simulink model "GFM_L_Filter_cc"  (R2016a)
settings: Solver=ode23tb  SolverMode=SingleTasking  StartTime=0.0  StopTime=Simulation_Time  FixedStep=Time_Step2  MaxStep=1e-5  RelTol=1e-3
PreLoadFcn:
  | GFM_L_Filter_Init;
InitFcn:
  | GFM_L_Filter_Init;
undefined symbols (not defined in the file): Chosen_Strategy, dur1, dur2, egfault, fb, GRD00_Lg, GRD00_Rg, Ib2, kd, Ki_cc_cp, Ki_Inertia_Less, Kp_cc_cp, kp_GFo, Kp_Inertia_Less, R, Sb, Start, Theta_Vvsc0, Time_Step, Time_Step2, Ug, Va0, Vb0, Vb1, Vb2, Vc0, Vm0, Vvsc0, wb, Zb
libraries: powerlib x25, Control_Lib x14, simulink x5, Source_Lib x1
(part 1 of 2)
settings Model: Creator=Frederic_Colas  LastModifiedBy=Frederic_Colas
settings DebuggingCC: UnconnectedInputMsg=none  UnconnectedOutputMsg=none  UnconnectedLineMsg=none  SFUnexpectedBacktrackingDiag=error  SFNoUnconditionalDefaultTransitionDiag=error
settings HardwareCC: ProdWordSize=32  ProdHWDeviceType=Specified
settings GRTTargetCC: TargetLangStandard=C99 (ISO)
settings ConfigComp: CovMetricSettings=dwe  CovSaveCumulativeToWorkspaceVar=off  CovSaveSingleToWorkspaceVar=off  CovExternalEMLEnable=on
settings SimscapeCC: SimscapeNormalizeSystem=off

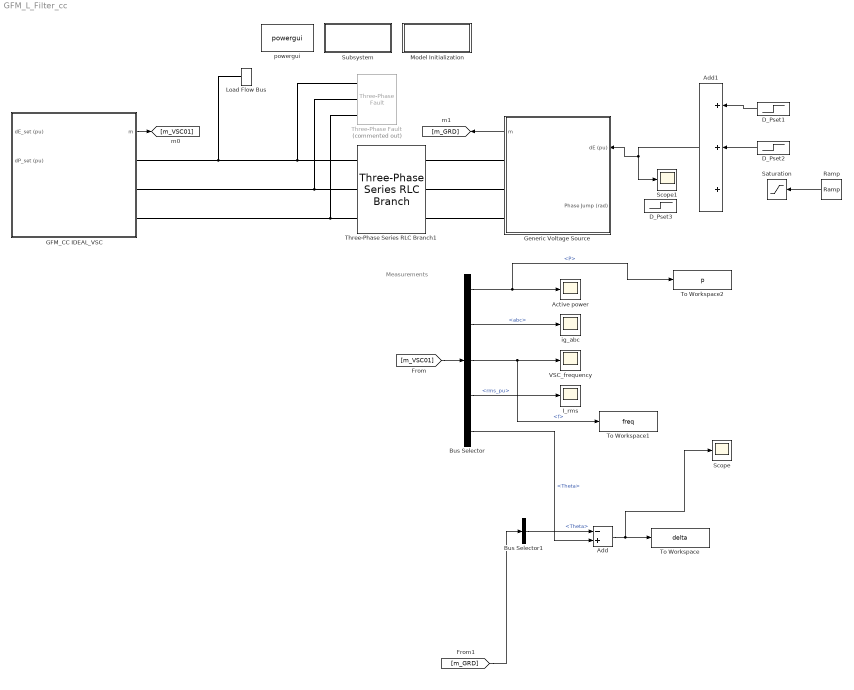
== system GFM_L_Filter_cc ==
  note: Measurements
  Active power : Scope
  Add : Sum  Inputs=-+
  Add1 : Sum  Inputs=+++
  Bus Selector : BusSelector  OutputSignals=P,Ig.abc,f,Ig.rms_pu,Theta
  Bus Selector1 : BusSelector  OutputSignals=Theta.Theta
  D_Pset1 : Step  Time=Start+0.1  After=-(1-egfault)  SampleTime=0
  D_Pset2 : Step  Time=Start+dur1+0.1  After=(1-egfault)  SampleTime=0
  D_Pset3 : Step  After=pi/6  SampleTime=0
  GFM_CC IDEAL_VSC : Subsystem  mask(VSC){fn=50, Sn=1000e6, Pn=1000e6, Udcn=640e3, Output_Delay=100e-6, Un1=320e3, Un2=400e3, Rt_pu=0.005, Lt_pu=0.15, Lm_pu=500, Rm_pu=500, DC_Link=Perfect DC Source, H_DC=inf, H_DC_sav=inf, wn_PLL=50, zeta_PLL=1, Val_Freq_Support=off, R_percent=4, dLc_pu=0.3, Rv=0.09, W_TVR=60, I_max_pu=1.2, Tr_I_max=10, Tau_fCC=0.01, wn_CC=1000, Kffi=on, Filtre_FF=off, w_ff=1000, Advanced=off, gainpopup=With Inertia, wn_Inertia_Less=5/(2*pi), Param_Inertia=PI, H_GFo=5, zeta_GFo=1, LFpopup=PV, P0=0.9, Q0=-0.069426, V0=1, Theta0=2.5991}
      mask prompts: fn "Nominal Frequency (Hz)"; Sn "Nominal Apparent Power (VA)"; Pn "Nominal Power (W)"; Udcn "Nominal DC Voltage (V)"; Output_Delay "Equivalent Output Delay (s)"; Un1 "VSC side Nominal Ph-Ph Voltage (V)"; Un2 "Grid side Nominal Ph-Ph Voltage (V)"; Rt_pu "R (pu)"; Lt_pu "L (pu)"; Lm_pu "Rm (pu)"; Rm_pu "Lm (pu)"; H_DC "DC inertia (ms)"; wn_PLL "Bandwidth (rad/s)"; zeta_PLL "Damping Ratio"; Val_Freq_Support "Frequency Support"; R_percent "Droop Gain (%)"; dLc_pu "Additional Virtual Impedance (pu)"; Rv "Damping Resistance (Rv)"; W_TVR "Dr filter"; I_max_pu "I max (pu)"; Tr_I_max "Current Loop time response (ms)"; Tau_fCC "Filter Time constant (s)"; wn_CC "Current Loop Bandwidth (rad/s))"; Kffi "Feedforward Enable"; Filtre_FF "Filter of ff enable"; w_ff "ff Filter Cutoff pulsation (rad/s)"; gainpopup "Strategy"; wn_Inertia_Less "Bandwidth (rad/s)"; H_GFo "Inertia H (s)"; zeta_GFo "Damping Ratio"; P0 "Initial Active Power (pu)"; Q0 "Initial Reactive Power (pu)"; V0 "Initial Voltage (pu)"; Theta0 "Initial Angle (°)"
      mask init:
      | Init_Base;
      | Init_VI;
      | Init_LF_L_modif;
      | Init_GFM_CC;
      settings: OpenFcn=|
      | NameStr = get_param(gcb,'Name');
      | open_system(gcbh, 'Mask');
      | 
      | h2AllOpenDlgs = DAStudio.ToolRoot.getOpenDialogs;
      | 
      | for i=1:length(h2AllOpenDlgs)
      |     try
      |          %disp(h2AllOpenDlgs(i).getSource.getBlock.Name);
      |         Dialog_block_name = h2AllOpenDlgs(i).getSource.getBlock.Name;
      |          %strcmp(Dialog_block_name, NameStr),
      |         if (strcmp(h2AllOpenDlgs(i).getSource.getBlock.Name, NameStr))
      |             iPos = h2AllOpenDlgs(i).position;
      |             h2AllOpenDlgs(i).position = [iPos(1)   iPos(2)   iPos(3)*1.4   iPos(4)];
      |         end
      |     end
      | end
      mask TypeOptions DC_Link: Perfect DC Source | No DC link capacitor | DC link capacitor
      mask Callback DC_Link:
      | % Get the mask parameter values. This is a cell
      | %   array of character vectors.
      | maskStr = get_param(gcb,'DC_Link');
      | p=Simulink.Mask.get(gcb);
      | 
      | % The pop-up menu is the first mask parameter.
      | %   Check the value selected in the pop-up
      | if strcmp(maskStr,'Perfect DC Source'),
      |     % Set the visibility of both parameters on when
      |     %   User-defined is selected in the pop-up.
      |     if strcmp(p.getParameter('H_DC').Visible,'on')
      |         p.getParameter('H_DC_sav').Value=p.getParameter('H_DC').Value;
      |     end
      |     p.getParameter('H_DC').Visible='off';
      |     p.getParameter('H_DC').Value='inf';
      | elseif strcmp(maskStr,'No DC link capacitor'),
      |     if strcmp(p.getParameter('H_DC').Visible,'on')
      |         p.getParameter('H_DC_sav').Value=p.getParameter('H_DC').Value;
      |     end
      |     p.getParameter('H_DC').Visible='off';
      |     p.getParameter('H_DC').Value='0';
      | else
      |     % Set the visibility of both parameters on when
      |     %   User-defined is selected in the pop-up.
      |     p.getParameter('H_DC').Visible='on';
      |     p.getParameter('H_DC').Value=p.getParameter('H_DC_sav').Value;
      | end
      mask Callback Advanced:
      | % Get the mask parameter values. This is a cell
      | %   array of character vectors.
      | maskStr = get_param(gcb,'Advanced');
      | p=Simulink.Mask.get(gcb);
      | 
      | % The pop-up menu is the first mask parameter.
      | %   Check the value selected in the pop-up
      | if strcmp(maskStr,'on'),
      | 
      |     % Set the visibility of both parameters on when
      |     %   User-defined is selected in the pop-up.
      |     %p.getDialogControl('TVR').Visible='on';
      |     %p.getDialogControl('TVI').Visible='on';
      |     %p.getDialogControl('LC_Filter').Visible='on';
      |     p.getDialogControl('Current_Sat').Visible='on';
      |     p.getDialogControl('CC').Visible='on';
      |     %p.getDialogControl('Param_Strat_3').Visible='off';
      | 
      | 
      | else
      | 
      |     % Set the visibility of both parameters on when
      |     %   User-defined is selected in the pop-up.
      |     %p.getDialogControl('TVR').Visible='off';
      |     %p.getDialogControl('TVI').Visible='off';
      |     %p.getDialogControl('LC_Filter').Visible='off';
      |     p.getDialogControl('Current_Sat').Visible='off';
      |     p.getDialogControl('CC').Visible='off';
      |     %p.getDialogControl('Param_Strat_3').Visible='off';
      | 
      | end
      mask TypeOptions gainpopup: Inertia Less | With Inertia
      mask Callback gainpopup:
      | % Get the mask parameter values. This is a cell
      | %   array of character vectors.
      | maskStr = get_param(gcb,'gainpopup');
      | p=Simulink.Mask.get(gcb);
      | 
      | % The pop-up menu is the first mask parameter.
      | %   Check the value selected in the pop-up
      | if strcmp(maskStr,'Inertia Less'),
      | 
      |     % Set the visibility of both parameters on when
      |     %   User-defined is selected in the pop-up.
      |     p.getDialogControl('No_Inertia').Visible='on';
      |     p.getDialogControl('Inertia').Visible='off';
      |     %p.getDialogControl('Param_Strat_3').Visible='off';
      | 
      | 
      | elseif strcmp(maskStr,'With Inertia'),
      | 
      |     % Set the visibility of both parameters on when
      |     %   User-defined is selected in the pop-up.
      |     p.getDialogControl('No_Inertia').Visible='off';
      |     p.getDialogControl('Inertia').Visible='on';
      |     %p.getDialogControl('Param_Strat_3').Visible='off';
      | 
      | 
      |     % Turn off the visibility of the Value field
      |     %   when User-defined is not selected.
      | 
      | else
      | 
      |     % Set the visibility of both parameters on when
      |     %   User-defined is selected in the pop-up.
      |     p.getDialogControl('No_Inertia').Visible='off';
      |     p.getDialogControl('Inertia').Visible='off';
      |     %p.getDialogControl('Param_Strat_3').Visible='off';
      | 
      | end
      mask TypeOptions Param_Inertia: VSM | PI
      mask TypeOptions LFpopup: Swing | PQ | PV
      mask Callback LFpopup:
      | % Get the mask parameter values. This is a cell
      | %   array of character vectors.
      | maskStr = get_param(gcb,'LFpopup');
      | p=Simulink.Mask.get(gcb);
      | 
      | % The pop-up menu is the first mask parameter.
      | %   Check the value selected in the pop-up
      | if strcmp(maskStr,'Swing'),
      | 
      |     % Set the visibility of both parameters on when
      |     %   User-defined is selected in the pop-up.
      |     p.getParameter('P0').Visible='off';
      |     p.getParameter('Q0').Visible='off';
      |     p.getParameter('V0').Visible='on';
      |     p.getParameter('Theta0').Visible='on';
      |     set_param([gcb '/Source_For_LF'],'BusType','swing');
      | 
      | elseif strcmp(maskStr,'PQ'),
      | 
      |     % Set the visibility of both parameters on when
      |     %   User-defined is selected in the pop-up.
      |     p.getParameter('P0').Visible='on';
      |     p.getParameter('Q0').Visible='on';
      |     p.getParameter('V0').Visible='off';
      |     p.getParameter('Theta0').Visible='off';
      |     set_param([gcb '/Source_For_LF'],'BusType','PQ');
      | 
      |     % Turn off the visibility of the Value field
      |     %   when User-defined is not selected.
      | else
      | 
      |     % Set the visibility of both parameters on when
      |     %   User-defined is selected in the pop-up.
      |     p.getParameter('P0').Visible='on';
      |     p.getParameter('Q0').Visible='off';
      |     p.getParameter('V0').Visible='on';
      |     p.getParameter('Theta0').Visible='off';
      |     set_param([gcb '/Source_For_LF'],'BusType','PV');
      | 
      | end
      mask DialogControl Container13 Prompt: PLL
      mask DialogControl Container14 Prompt: Frequency Support
      mask DialogControl VI Prompt: Virtual Impedance
      mask DialogControl TVR Prompt: Transient Virtual Resistor
      mask DialogControl Current_Sat Prompt: Current Limitation
      mask DialogControl CC Prompt: Current Loop
      mask DialogControl Control4 Prompt: Initial Operating Point
      mask DialogControl Container24 Prompt: VSC side
      mask DialogControl LF_vsc_str Prompt: V0 = 1.0552 pu, Angle = 25.2352°
      mask DialogControl Container25 Prompt: PCC
      mask DialogControl UpdateLoadflow Prompt: Update Loadflow
      mask DialogControl UpdateLoadflow Callback: LoadFlow_VSC
      mask Display:
      | x1=0.05;
      | y1=0.2;
      | %
      | plot([0.5 0.5]+x1,[0.97,0.8]-y1)
      | plot([0.5 0.32]+x1,[0.80 0.71]-y1)
      | plot([0.32 0.32]+x1,[0.80 0.52]-y1)
      | plot([0.32 0.5]+x1,[0.62 0.52]-y1)
      | plot([0.5 0.5]+x1,[0.52 0.35]-y1)
      | plot([0.45 0.5 0.43]+x1,[0.59 0.52 0.51]-y1)
      | %
      | plot([0.28 0.28]+x1,[0.74 0.58]-y1)
      | plot([0.28 0.20]+x1,[0.66 0.66]-y1)
      | %
      | plot([0.5 0.63]+x1,[0.84 0.84]-y1)
      | plot([0.63 0.63]+x1,[0.84 0.72]-y1)
      | plot([0.63 0.59]+x1,[0.72 0.65]-y1)
      | plot([0.63 0.67]+x1,[0.72 0.65]-y1)
      | plot([0.59 0.67]+x1,[0.65 0.65]-y1)
      | plot([0.63 0.63]+x1,[0.65 0.47]-y1)
      | plot([0.5 0.63]+x1,[0.47 0.47]-y1)
      | plot([0.58 0.67]+x1,[0.72 0.72]-y1)
      | %
      | color('blue')
      | text(0.3,0.10,'L-Filter GFM CC')
      | 
      | port_label('input',1,'\DeltaE (pu)','texmode','on');
      | port_label('input',2,'\DeltaP (pu)','texmode','on');
      | port_label('output',1,'m');
      | port_label('rconn',1,'A');
      | port_label('rconn',2,'B');
      | port_label('rconn',3,'C');
      | port_label('lconn',1,'+');
      | port_label('lconn',2,'-');
  Generic Voltage Source : Subsystem  AncestorBlock=Source_Lib/Generic Voltage Source  mask(GenericVoltageSource){SourceNature_str=INFINITE, fn=50, Sn=1e9, Un=Ug, H_s=5, DroopOnOff=on, R_percent=4, TN=1, TD=2, Time_Step=Time_Step, LFpopup=Swing, P0=-0.89593, Q0=0.11017, V0=1, Theta0=0}
      mask prompts: SourceNature_str "Nature of the voltage source"; fn "Nominal frequency fn [Hz]"; Sn "Nominal apparent power Sn [VA]"; Un "Nominal voltage Un [V RMS Ph2Ph]"; H_s "Inertia H [s]"; DroopOnOff "Frequency DROOP activation"; R_percent "Droop gain Kp [%]"; TN "Network time constant Lead [s]"; TD "Network time constant Lag [s]"; Time_Step "Output Delay (s)"; P0 "Active power P0 (pu)"; Q0 "Reactive power Q0 (pu)"; V0 "Initial Voltage (pu)"; Theta0 "Initial angle (°)"
      mask init:
      | % Update Name of LF bus for internal purpose
      | NameStr = [get_param(gcb,'Name')];% '_LF'];
      | set_param([gcb '/Load Flow Bus'],'ID',NameStr);  
      | 
      | % Base specification
      | fb = fn;                % [Hz] base frequency
      | Sb = Sn;                % [VA] base power
      | Ub = Un;                % [V] base ph2ph voltage
      | Vb = Un/sqrt(3);        % [V] base ph2N voltage
      | Ib = Sb/(3*Vb);         % [A] base current
      | Zb = Vb*Ib;             % [Ohm] base impedance
      | 
      | % Set the frequency droop gain
      | R = R_percent / 100;
      | 
      | %Initialize correctly the LoadFlow bus parameters connected to PCC
      |     VLF = V0;
      |     ThetaLF = Theta0;
      |     if (LFpopup == 'PQ')
      |         VLF = 1;
      |         ThetaLF = 0;
      |     elseif (LFpopup == 'PV')
      |         VLF = V0;
      |         ThetaLF = 0;        
      |     end
      |     set_param([gcb '/Load Flow Bus'],'Vref',num2str(VLF),'Vangle',num2str(ThetaLF));
      | 
      | 
      | % Update mask display:
      | % mo = get_param(gcb,'MaskObject');
      | % Generate string to display LF results on Mask
      |     mo = get_param(gcb,'MaskObject');
      |     mo.getDialogControl('LF_pcc_str').Prompt = ['V0 = ', num2str(V0),' pu, Angle = ', num2str(Theta0),'°'];
      |     mo.getDialogControl('LF_pcc_Power_str').Prompt = ['P0 = ', num2str(P0),' pu, Q0 = ', num2str(Q0),' pu'];
      mask TypeOptions SourceNature_str: INFINITE | INERTIAL
      mask Callback SourceNature_str:
      | % Get the mask parameter values. This is a cell
      | %   array of character vectors.
      | maskStr = get_param(gcb,'SourceNature_str');
      | p=Simulink.Mask.get(gcb);
      | 
      | % The pop-up menu is the first mask parameter.
      | %   Check the value selected in the pop-up
      | if strcmp(maskStr,'INFINITE')
      |     p.getDialogControl('Inertial').Visible='off';
      |    %p.getParameter('H_s').Visible='off';
      |    %p.getParameter('DroopOnOff').Visible='off';
      |    %DroopOnOff = 'off';
      |    %p.getParameter('R_percent').Visible='off';
      |    %p.getParameter('TN').Visible='off';
      |    %p.getParameter('TD').Visible='off';
      |    set_param([gcb '/SourceNature'],'Value','1')
      | else
      |    %p.getParameter('H_s').Visible='on';
      |    %p.getParameter('DroopOnOff').Visible='on';
      |    %DroopOnOff = 'on';
      |    %p.getParameter('R_percent').Visible='on';
      |    %p.getParameter('TN').Visible='on';
      |    %p.getParameter('TD').Visible='on';
      |    p.getDialogControl('Inertial').Visible='on';
      |    set_param([gcb '/SourceNature'],'Value','2')
      | end
      mask Callback DroopOnOff:
      | % Get the mask parameter values. This is a cell
      | %   array of character vectors.
      | maskStr = get_param(gcb,'DroopOnOff');
      | p=Simulink.Mask.get(gcb);
      | 
      | if strcmp(maskStr,'on'),
      |     p.getParameter('R_percent').Enabled='on';
      | else
      |     p.getParameter('R_percent').Enabled='off';
      | end
      mask TypeOptions LFpopup: Swing | PQ | PV
      mask Callback LFpopup:
      | % Get the mask parameter values. This is a cell
      | %   array of character vectors.
      | maskStr = get_param(gcb,'LFpopup');
      | p=Simulink.Mask.get(gcb);
      | 
      | % The pop-up menu is the first mask parameter.
      | %   Check the value selected in the pop-up
      | if strcmp(maskStr,'Swing'),
      | 
      |     % Set the visibility of both parameters on when
      |     %   User-defined is selected in the pop-up.
      |     p.getParameter('P0').Visible='off';
      |     p.getParameter('Q0').Visible='off';
      |     p.getParameter('V0').Visible='on';
      |     p.getParameter('Theta0').Visible='on';
      |     set_param([gcb '/Source_For_LF'],'BusType','swing');
      | 
      | elseif strcmp(maskStr,'PQ'),
      | 
      |     % Set the visibility of both parameters on when
      |     %   User-defined is selected in the pop-up.
      |     p.getParameter('P0').Visible='on';
      |     p.getParameter('Q0').Visible='on';
      |     p.getParameter('V0').Visible='off';
      |     p.getParameter('Theta0').Visible='off';
      |     set_param([gcb '/Source_For_LF'],'BusType','PQ');
      | 
      |     % Turn off the visibility of the Value field
      |     %   when User-defined is not selected.
      | else
      | 
      |     % Set the visibility of both parameters on when
      |     %   User-defined is selected in the pop-up.
      |     p.getParameter('P0').Visible='on';
      |     p.getParameter('Q0').Visible='off';
      |     p.getParameter('V0').Visible='on';
      |     p.getParameter('Theta0').Visible='off';
      |     set_param([gcb '/Source_For_LF'],'BusType','PV');
      | 
      | end
      mask DialogControl Control1 Prompt: Initial Operating Point
      mask DialogControl Container6 Prompt: PCC
      mask DialogControl Control4 Prompt: Update Loadflow
      mask DialogControl Control4 Callback: LoadFlow_VSC
      mask Display:
      | if (SourceNature_str == 1)
      |     image(imread('infinite.png'));
      |     color('blue')
      |     text(0.3,0.10,'Infinite bus')
      | else
      |     image(imread('inertia.png'));
      |     color('blue')
      |     text(0.3,0.10,'Inertia Emulation')
      | end
      | 
      | port_label('input',1,'\DeltaE (pu)','texmode','on');
      | port_label('input',2,'\Delta\theta (rad)','texmode','on');
      | port_label('output',1,'m');
      | port_label('rconn',1,'A');
      | port_label('rconn',2,'B');
      | port_label('rconn',3,'C');
  I_rms : Scope
  Load Flow Bus : powerlib/Measurements/Load Flow Bus  LConnTagsString=a  Phases=single  Connectors=on one side  ID=BUS_1  Vbase=Ug  Vref=1  Vangle=0  VLF=1  VLFb=1  VLFc=1  angleLF=2.599  angleLFb=0  angleLFc=0
  Model Initialization : Subsystem  mask(Model Functions){InitFcnX=GFM_L_Filter_Init;, prel=on, posl=off, inif=on, strf=off}
      mask prompts: InitFcnX "Initialisation"; prel "Preload Function"; posl "PostLoad Function"; inif "InitFcn"; strf "StartFcn"
      mask init:
      | currentBlock = gcb;
      | root = bdroot(currentBlock);
      | 
      | if ~strcmp(get_param(root,'BlockDiagramType'),'library')
      |     if prel==1
      |         set_param(root, 'PreLoadFcn', InitFcnX);
      |     else
      |         set_param(root, 'PreLoadFcn', '');
      |     end
      |     if inif==1
      |         set_param(root, 'InitFcn', InitFcnX);
      |     else
      |         set_param(root, 'InitFcn', '');
      |     end
      |     if strf==1
      |         set_param(root, 'StartFcn', InitFcnX);
      |     else
      |         set_param(root, 'StartFcn', '');
      |     end
      |     if posl==1
      |         set_param(root, 'PostLoadFcn', InitFcnX);
      |     else
      |         set_param(root, 'PostLoadFcn', '');
      |     end
      | end
      | 
      | pos = get_param(currentBlock, 'Position');
      | width = pos(3) - pos(1); height = pos(4) - pos(2);
      | txt = [ upper(root) '\n' '- InitFcn. . . . . '  get_param(root, 'InitFcn') ];
      settings: CopyFcn=set_param(gcb,'LinkStatus','none')
      mask Display:
      | %text(5, height*0.5, txt, 'horizontalAlignment', 'left', 'verticalAlignment', 'middle') ;
      | color('blue'),disp('Initialization Function\nParameters')
  Ramp : simulink/Sources/Ramp  slope=(1-egfault)/(dur2)  start=Start+dur1+0.1  X0=0
  Saturation : Saturate  UpperLimit=1-egfault  LowerLimit=0
  Scope : Scope
  Scope1 : Scope
  Subsystem : Subsystem
      settings: OpenFcn=LoadFlow_VSC
      mask Display: color('blue'),disp('Update Loadflow')
  Three-Phase Series RLC Branch1 : powerlib/Elements/Three-Phase Series RLC Branch  LConnTagsString=A|B|C  RConnTagsString=A|B|C  BranchType=RL  Resistance=GRD00_Rg  Inductance=GRD00_Lg  Capacitance=1e-6  Measurements=None
  Three-Phase Fault : powerlib/Elements/Three-Phase Fault  Commented=on  InitialStates=0  FaultA=on  FaultB=on  FaultC=on  GroundFault=on  SwitchTimes=[0.2 0.4]  External=off  SwitchStatus=NaN  FaultResistance=0.001  GroundResistance=0.01  SnubberResistance=1e6  SnubberCapacitance=inf  Measurements=None
  To Workspace : ToWorkspace  VariableName=delta  SaveFormat=Timeseries  SampleTime=Time_Step
  To Workspace1 : ToWorkspace  VariableName=freq  SaveFormat=Timeseries  SampleTime=Time_Step
  To Workspace2 : ToWorkspace  VariableName=p  SaveFormat=Timeseries  SampleTime=Time_Step
  VSC_frequency : Scope
  ig_abc : Scope
  powergui : powerlib/powergui  Priority=1  SimulationMode=Discrete  SampleTime=Time_Step2  frequency=60  Iterations=50  frequencyindice=50  Pbase=1000000000  ErrMax=1e-6  UnitsV=kV  UnitsW=MW  buscounter=0  FunctionMessages=off  echomessages=off  EnableUseOfTLC=off  CurrentSourceSwitches=off  DisableSnubberDevices=off  DisableRonSwitches=off  DisableVfSwitches=off  DisplayEquations=off  AutomaticDiscreteSolvers=off  SolverType=Tustin/Backward Euler (TBE)  Interpol=off  ExternalGateDelay=off  methode=off  Ts=100  x0status=blocks  SPID=on  SwTol=0  HookPort=off  NonlinearTolerance=1e-4  nMaxIteration=100  ContinueOnMaxIteration=off  RestoreLinks=warning  ResistiveCurrentMeasurement=off  Frange=[0:2:500]  Ylog=off  Xlog=on  ShowGrid=off  save=off  variable=ZData  structure=0  ZoomFFT=off  StartTime=0.0  cycles=1  DisplayStyle=1  fundamental=60  FreqAxis=off  MaxFrequency=1000  frequencyindicesteady=1  RmsSteady=1  display=off
  wires:
  [m_VSC01] -> Bus Selector/1
  Bus Selector/1 -> To Workspace2/1, Active power/1  "<P>"
  Bus Selector/4 -> I_rms/1  "<rms_pu>"
  Bus Selector/2 -> ig_abc/1  "<abc>"
  Bus Selector/3 -> VSC_frequency/1, To Workspace1/1  "<f>"
  GFM_CC IDEAL_VSC/1(m) -> [m_VSC01]
  Generic Voltage Source/1(m) -> [m_GRD]
  [m_GRD] -> Bus Selector1/1
  Bus Selector1/1 -> Add/1  "<Theta>"
  Bus Selector/5 -> Add/2  "<Theta>"
  Add/1 -> Scope/1, To Workspace/1
  D_Pset1/1 -> Add1/1
  Ramp/1 -> Saturation/1
  D_Pset2/1 -> Add1/2
  Add1/1 -> Generic Voltage Source/1(dE (pu)), Scope1/1
  connections:
  Load Flow Bus/LConn1 -- Three-Phase Fault/LConn1 -- Three-Phase Series RLC Branch1/LConn1 -- GFM_CC IDEAL_VSC/RConn1
  GFM_CC IDEAL_VSC/RConn3 -- Three-Phase Fault/LConn3 -- Three-Phase Series RLC Branch1/LConn3
  GFM_CC IDEAL_VSC/RConn2 -- Three-Phase Fault/LConn2 -- Three-Phase Series RLC Branch1/LConn2
  Generic Voltage Source/RConn1 -- Three-Phase Series RLC Branch1/RConn1
  Generic Voltage Source/RConn2 -- Three-Phase Series RLC Branch1/RConn2
  Generic Voltage Source/RConn3 -- Three-Phase Series RLC Branch1/RConn3

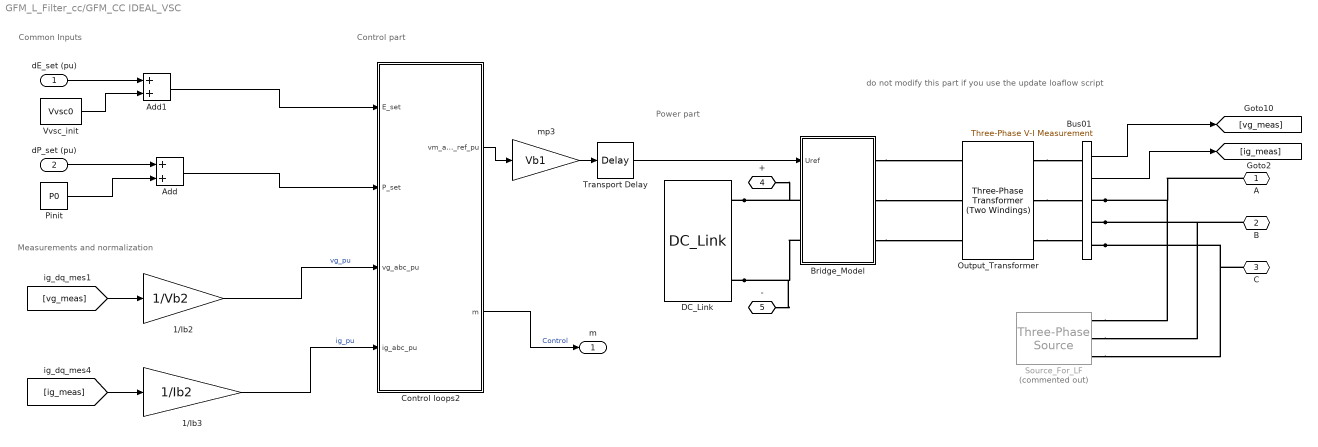
== system GFM_L_Filter_cc/GFM_CC IDEAL_VSC ==
  note: Control part
  note: Measurements and normalization
  note: Power part
  note: Common Inputs
  note: do not modify this part if you use the update loaflow script
  dE_set (pu) : Inport
  dP_set (pu) : Inport  Port=2
  1/Ib2 : Gain  Gain=1/Vb2
  1/Ib3 : Gain  Gain=1/Ib2
  Add : Sum
  Add1 : Sum
  Bridge_Model : Subsystem
  Bus01 : powerlib/Measurements/Three-Phase V-I Measurement  VoltageMeasurement=phase-to-ground  SetLabelV=off  LabelV=Vabc  Vpu=off  VpuLL=off  CurrentMeasurement=yes  SetLabelI=off  LabelI=Iabc  Ipu=off  Pbase=100e6  Vbase=500e3  OutputType=Complex  PhasorSimulation=off  PSBequivalent=0
  Control loops2 : Subsystem
  DC_Link : Source_Lib/DC_Link  Udc=Udcn  Pb=Pn  H_DC=H_DC
  Output_Transformer : powerlib/Elements/Three-Phase Transformer (Two Windings)  Winding1Connection=Yg  Winding2Connection=Yg  CoreType=Three single-phase transformers  SetSaturation=off  Hysteresis=off  DataFile='hysteresis'  SetInitialFlux=off  Measurements=None  UNITS=pu  NominalPower=[Sn , fb]  Winding1=[Un1 , Rt_pu/2 , Lt_pu/2]  Winding2=[Un2 , Rt_pu/2 , Lt_pu/2]  Rm=Rm_pu  Lm=Lm_pu  L0=0.5  Saturation=[ 0,0 ; 0.0024,1.2 ; 1.0,1.52 ]  InitialFluxes=[ 0.8 , -0.8 , 0.7 ]  BreakLoop=off  DiscreteSolver=Trapezoidal iterative  DataType=off  TransfoNumber=1
  Pinit : Constant  Value=P0
  Source_For_LF : powerlib/Electrical Sources/Three-Phase Source  Commented=on  InternalConnection=Yg  VoltagePhases=off  Voltage=(400000)*1  PhaseAngle=2.5991  Voltage_phases=[25e3 25e3 25e3]/sqrt(3)  PhaseAngles_phases=[0 -120 +120]  Frequency=fb  NonIdealSource=off  SpecifyImpedance=off  Resistance=0  Inductance=0  ShortCircuitLevel=100e6  BaseVoltage=Un  XRratio=7  BusType=PV  Pref=P0*Sb  Qref=Q0*Sb  Prefabc=[10e3, 10e3, 10e3]  Qrefabc=[0, 0, 0]  Qmin=-inf  Qmax=inf
  Transport Delay : TransportDelay  DelayTime=Output_Delay  InitialOutput=[Va0 Vb0 Vc0]
  Vvsc_init : Constant  Value=Vvsc0
  mp3 : Gain  Gain=Vb1
  A : PMIOPort  Side=Right
  B : PMIOPort  Port=2  Side=Right
  C : PMIOPort  Port=3  Side=Right
  + : PMIOPort  Port=4  Side=Left
  - : PMIOPort  Port=5  Side=Left
  m : Outport
  wires:
  [ig_meas] -> 1/Ib3/1
  Bus01/2 -> [ig_meas]
  dE_set (pu)/1 -> Add1/1
  Bus01/1 -> [vg_meas]
  Vvsc_init/1 -> Add1/2
  Pinit/1 -> Add/2
  dP_set (pu)/1 -> Add/1
  Transport Delay/1 -> Bridge_Model/1(Uref)
  Add1/1 -> Control loops2/1(E_set)
  Control loops2/1(vm_abc_ref_pu) -> mp3/1
  [vg_meas] -> 1/Ib2/1
  1/Ib2/1 -> Control loops2/3(vg_abc_pu)  "vg_pu"
  1/Ib3/1 -> Control loops2/4(ig_abc_pu)  "ig_pu"
  mp3/1 -> Transport Delay/1
  Control loops2/2(m) -> m/1  "Control"
  Add/1 -> Control loops2/2(P_set)
  connections:
  DC_Link/RConn3 -- -/RConn1 -- Bridge_Model/LConn2
  DC_Link/RConn1 -- +/RConn1 -- Bridge_Model/LConn1
  Bus01/RConn3 -- C/RConn1 -- Source_For_LF/RConn3
  Bus01/RConn1 -- A/RConn1 -- Source_For_LF/RConn1
  Bridge_Model/RConn3 -- Output_Transformer/LConn3
  Bridge_Model/RConn2 -- Output_Transformer/LConn2
  Bridge_Model/RConn1 -- Output_Transformer/LConn1
  Bus01/RConn2 -- B/RConn1 -- Source_For_LF/RConn2
  Output_Transformer/RConn3 -- Bus01/LConn3
  Output_Transformer/RConn2 -- Bus01/LConn2
  Output_Transformer/RConn1 -- Bus01/LConn1

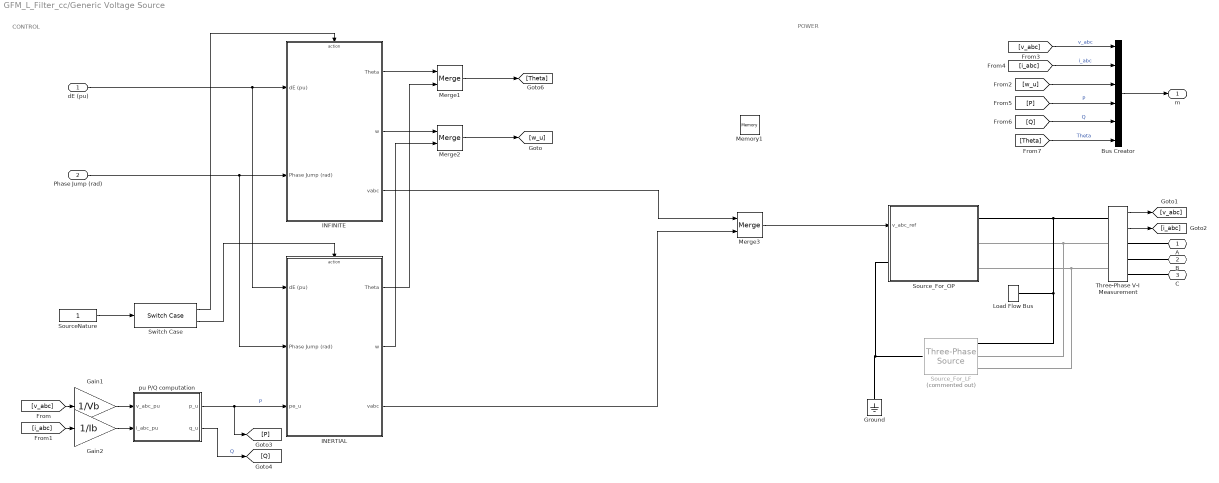
== system GFM_L_Filter_cc/Generic Voltage Source ==
  note: CONTROL
  note: POWER
  dE (pu) : Inport
  Phase Jump (rad) : Inport  Port=2
  " pu P/Q computation" : Subsystem  DialogController=POWERSYS.PowerSysDialog
  Bus Creator : BusCreator  Inputs=6
  Gain1 : Gain  Gain=1/Vb
  Gain2 : Gain  Gain=1/Ib
  Ground : powerlib/Elements/Ground  LConnTagsString=a
  INERTIAL : Subsystem
  INFINITE : Subsystem
  Load Flow Bus : powerlib/Measurements/Load Flow Bus  LConnTagsString=a  Phases=single  Connectors=on one side  ID=Generic Voltage Source  Vbase=Un  Vref=1  Vangle=0  VLF=1  VLFb=1  VLFc=1  angleLF=0  angleLFb=0  angleLFc=0
  Memory1 : Memory
  Merge1 : Merge
  Merge2 : Merge
  Merge3 : Merge
  SourceNature : Constant
  Source_For_LF : powerlib/Electrical Sources/Three-Phase Source  Commented=on  InternalConnection=Yn  VoltagePhases=off  Voltage=(400000)*1  PhaseAngle=0  Voltage_phases=[25e3 25e3 25e3]/sqrt(3)  PhaseAngles_phases=[0 -120 +120]  Frequency=fb  NonIdealSource=off  SpecifyImpedance=off  Resistance=0  Inductance=0  ShortCircuitLevel=100e6  BaseVoltage=Un  XRratio=7  BusType=swing  Pref=P0*Sb  Qref=Q0*Sb  Prefabc=[10e3, 10e3, 10e3]  Qrefabc=[0, 0, 0]  Qmin=-inf  Qmax=inf
  Source_For_OP : Subsystem
  Switch Case : SwitchCase  CaseConditions={1, 2}  ShowDefaultCase=off
  Three-Phase V-I Measurement : powerlib/Measurements/Three-Phase V-I Measurement  VoltageMeasurement=phase-to-ground  SetLabelV=off  LabelV=v_abc  Vpu=off  VpuLL=off  CurrentMeasurement=yes  SetLabelI=off  LabelI=i_abc  Ipu=off  Pbase=100e6  Vbase=500e3  OutputType=Complex  PhasorSimulation=off  PSBequivalent=0
  A : PMIOPort  Side=Right
  B : PMIOPort  Port=2  Side=Right
  C : PMIOPort  Port=3  Side=Right
  m : Outport
  wires:
  INERTIAL/3(vabc) -> Merge3/2
  INFINITE/3(vabc) -> Merge3/1
  Merge3/1 -> Source_For_OP/1(v_abc_ref)
  Merge2/1 -> [w_u]
  INERTIAL/2(w) -> Merge2/2
  INFINITE/2(w) -> Merge2/1
  INERTIAL/1(Theta) -> Merge1/2
  Phase Jump (rad)/1 -> INFINITE/2(Phase Jump (rad)), INERTIAL/2(Phase Jump (rad))
  dE (pu)/1 -> INFINITE/1(dE (pu)), INERTIAL/1(dE (pu))
  Merge1/1 -> [Theta]
  INFINITE/1(Theta) -> Merge1/1
  [Theta] -> Bus Creator/6  "Theta"
  SourceNature/1 -> Switch Case/1
  Switch Case/1 -> INFINITE/Action
  Switch Case/2 -> INERTIAL/Action
  [v_abc] -> Gain1/1
  [i_abc] -> Gain2/1
  Gain1/1 -> " pu P/Q computation"/1(v_abc_pu)
  Gain2/1 -> " pu P/Q computation"/2(i_abc_pu)
  " pu P/Q computation"/2(q_u) -> [Q]  "Q"
  " pu P/Q computation"/1(p_u) -> [P], INERTIAL/3(pe_u)  "P"
  [v_abc] -> Bus Creator/1  "v_abc"
  [i_abc] -> Bus Creator/2  "i_abc"
  [w_u] -> Bus Creator/3
  Bus Creator/1 -> m/1
  Three-Phase V-I Measurement/1 -> [v_abc]
  Three-Phase V-I Measurement/2 -> [i_abc]
  [P] -> Bus Creator/4  "P"
  [Q] -> Bus Creator/5  "Q"
  connections:
  Source_For_LF/RConn2 -- Three-Phase V-I Measurement/LConn2 -- Source_For_OP/RConn2
  Source_For_OP/LConn1 -- Ground/LConn1
  Source_For_LF/RConn3 -- Three-Phase V-I Measurement/LConn3 -- Source_For_OP/RConn3
  Source_For_OP/RConn1 -- Source_For_LF/RConn1 -- Load Flow Bus/LConn1 -- Three-Phase V-I Measurement/LConn1
  Three-Phase V-I Measurement/RConn1 -- A/RConn1
  Three-Phase V-I Measurement/RConn2 -- B/RConn1
  Three-Phase V-I Measurement/RConn3 -- C/RConn1

== system GFM_L_Filter_cc/Model Initialization ==

== system GFM_L_Filter_cc/Subsystem ==

== system GFM_L_Filter_cc/GFM_CC IDEAL_VSC/Bridge_Model ==
  Uref : Inport
  NOT1 : Logic  Operator=NOT  IconShape=distinctive  AllPortsSameDT=off  OutDataTypeStr=boolean
  Saturation : Saturate  UpperLimit=1  LowerLimit=-1
  Step : Step  Time=Output_Delay  SampleTime=0
  Three-Phase Breaker1 : powerlib/Elements/Three-Phase Breaker  InitialState=closed  SwitchA=on  SwitchB=on  SwitchC=on  SwitchTimes="[4/60  10/60]"  External=on  BreakerResistance=1e-5*Zb  SnubberResistance=1e6  SnubberCapacitance=inf  Measurements=None
  Three-Phase Breaker2 : powerlib/Elements/Three-Phase Breaker  InitialState=open  SwitchA=on  SwitchB=on  SwitchC=on  SwitchTimes="[4/60  10/60]"  External=on  BreakerResistance=1e-5*Zb  SnubberResistance=1e6  SnubberCapacitance=inf  Measurements=None
  Three-Phase Source : powerlib/Electrical Sources/Three-Phase Source  InternalConnection=Yg  VoltagePhases=off  Voltage=Vm0*Un1  PhaseAngle=Theta_Vm0  Voltage_phases=[25e3 25e3 25e3]/sqrt(3)  PhaseAngles_phases=[0 -120 +120]  Frequency=fb  NonIdealSource=off  SpecifyImpedance=off  Resistance=0  Inductance=0  ShortCircuitLevel=100e6  BaseVoltage=VSC01_Un1  XRratio=7  BusType=swing  Pref=0.3  Qref=0  Prefabc=[10e3, 10e3, 10e3]  Qrefabc=[0, 0, 0]  Qmin=-Inf  Qmax=Inf
  Universal Bridge : powerlib/Power Electronics/Universal Bridge  Arms=3  SnubberResistance=1e5  SnubberCapacitance=inf  Device=Average-model based VSC  Ron=1e-3  Lon=0  ForwardVoltages="[  0  0  ]"  ForwardVoltage=0  GTOparameters=[ 10e-6 , 20e-6 ]  IGBTparameters=[ 1e-6 , 2e-6 ]  Measurements=None  Measurements_2=None  converterType=Rectifier
  mp3 : Gain  Gain=2/Udcn
  PhA : PMIOPort  Side=Right
  PhB : PMIOPort  Port=2  Side=Right
  PhC : PMIOPort  Port=3  Side=Right
  Vdc+ : PMIOPort  Port=4  Side=Left
  Vdc- : PMIOPort  Port=5  Side=Left
  wires:
  Uref/1 -> mp3/1
  mp3/1 -> Saturation/1
  Step/1 -> NOT1/1, Three-Phase Breaker2/1
  NOT1/1 -> Three-Phase Breaker1/1
  Saturation/1 -> Universal Bridge/1
  connections:
  Universal Bridge/RConn2 -- Vdc-/RConn1
  Universal Bridge/RConn1 -- Vdc+/RConn1
  Three-Phase Source/RConn3 -- Three-Phase Breaker1/RConn3
  Three-Phase Source/RConn2 -- Three-Phase Breaker1/RConn2
  Three-Phase Source/RConn1 -- Three-Phase Breaker1/RConn1
  Three-Phase Breaker2/RConn3 -- Universal Bridge/LConn3
  Three-Phase Breaker2/RConn2 -- Universal Bridge/LConn2
  Three-Phase Breaker2/RConn1 -- Universal Bridge/LConn1
  PhC/RConn1 -- Three-Phase Breaker1/LConn3 -- Three-Phase Breaker2/LConn3
  PhB/RConn1 -- Three-Phase Breaker1/LConn2 -- Three-Phase Breaker2/LConn2
  PhA/RConn1 -- Three-Phase Breaker1/LConn1 -- Three-Phase Breaker2/LConn1

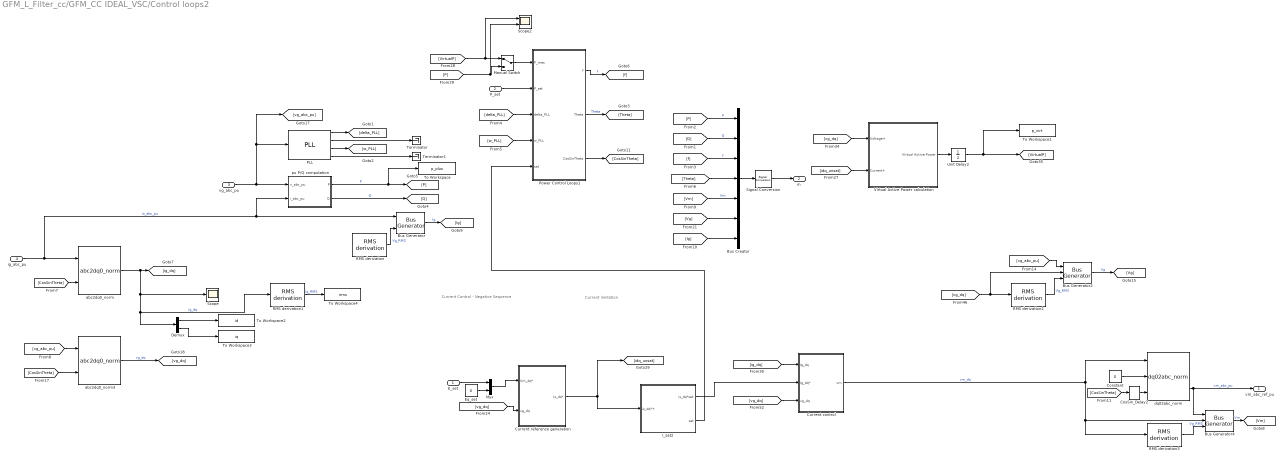
== system GFM_L_Filter_cc/GFM_CC IDEAL_VSC/Control loops2 ==
  note: Current Control - Negative Sequence
  note: Current limitation
  E_set : Inport
  P_set : Inport  Port=2
  vg_abc_pu : Inport  Port=3
  ig_abc_pu : Inport  Port=4
  " pu P/Q computation" : Subsystem  DialogController=POWERSYS.PowerSysDialog
  Bus Creator : BusCreator  Inputs=7
  Bus Generator : Control_Lib/Bus Generator  Gpu=Ib2
  Bus Generator2 : Control_Lib/Bus Generator  Gpu=Vb2
  Bus Generator4 : Control_Lib/Bus Generator  Gpu=Vb1
  Constant : Constant  Value=0
  CosSin_Delay2 : Control_Lib/CosSin_Delay  dTheta=wb*(Output_Delay)
  Current control : Subsystem  AncestorBlock=GFM_Lib/GFM_CC IDEAL_VSC/Control loops/Current control
  Current reference generation : Subsystem  mask{Tau_fCC=0.01, Lt=Lt_pu}
      mask prompts: Tau_fCC "Tau_f"; Lt "Model impedance"
  Demux : Demux  Outputs=2
  Eq_set : Constant  Value=0
  I_sat2 : Subsystem  mask{I_sat=I_max_pu}
      mask prompts: I_sat "Isat( pu)"
  Manual Switch : ManualSwitch
  Mux : Mux  Inputs=2
  PLL : Control_Lib/PLL  fb=fb  wn_PLL=wn_PLL  zeta_PLL=zeta_PLL  Theta0=Theta0
  Power Control Loops1 : Subsystem  AncestorBlock=Control_Lib/Power Control Loops  mask{Theta0_VSC=Theta_Vvsc0}
      mask prompts: Theta0_VSC "Initial VSC angle"
      mask DialogControl DescGroupVar Prompt: Parameters
  RMS derivation{,1..3} (4 alike) : Control_Lib/RMS derivation  SystemSampleTime=-1  Latency=0  AutoFrameSizeCalculation=off
  Scope : Scope
  Scope2 : Scope  NumInputPorts=2
  Signal Conversion : SignalConversion  OverrideOpt=off
  Terminator : Terminator
  Terminator1 : Terminator
  To Workspace : ToWorkspace  VariableName=p_plus  SaveFormat=Timeseries  SampleTime=-1
  To Workspace1 : ToWorkspace  VariableName=p_virt  SaveFormat=Timeseries  SampleTime=-1
  To Workspace2 : ToWorkspace  VariableName=id  SaveFormat=Timeseries  SampleTime=Time_Step
  To Workspace3 : ToWorkspace  VariableName=iq  SaveFormat=Timeseries  SampleTime=Time_Step
  To Workspace4 : ToWorkspace  VariableName=irms  SaveFormat=Timeseries  SampleTime=Time_Step
  Unit Delay2 : UnitDelay  InitialCondition=P0  SampleTime=-1  HasFrameUpgradeWarning=on
  Virtual Active Power calculation : Subsystem
  abc2dq0_norm : Control_Lib/abc2dq0_norm  referenceAxisMode=Reference axis at 90 degrees behind phase_a  baseUpdateGain=1/sqrt(3)
  abc2dq0_norm3 : Control_Lib/abc2dq0_norm  referenceAxisMode=Reference axis at 90 degrees behind phase_a  baseUpdateGain=1/sqrt(3)
  dq02abc_norm : Control_Lib/dq02abc_norm  referenceAxisMode=Reference axis at 90 degrees behind phase_a  baseUpdateGain=sqrt(3)
  vm_abc_ref_pu : Outport  PortDimensions=3
  m : Outport  Port=2
  wires:
  [Ig] -> Bus Creator/7
  [Vg] -> Bus Creator/6
  RMS derivation3/1 -> Bus Generator4/3  "Vg_RMS"
  Bus Generator4/1 -> [Vm]  "Vm"
  [CosSinTheta] -> abc2dq0_norm3/2
  [vg_abc_pu] -> abc2dq0_norm3/1
  abc2dq0_norm3/2 -> [vg_dq]  "vg_dq"
  [vg_abc_pu] -> Bus Generator2/1
  RMS derivation2/1 -> Bus Generator2/3  "Vg_RMS"
  Bus Generator2/1 -> [Vg]  "Vg"
  RMS derivation/1 -> Bus Generator/3  "Vg_RMS"
  CosSin_Delay2/1 -> dq02abc_norm/3
  PLL/4 -> Terminator1/1
  PLL/2 -> Terminator/1
  Constant/1 -> dq02abc_norm/2
  Power Control Loops1/3(CosSinTheta) -> [CosSinTheta]
  PLL/3 -> [w_PLL]
  PLL/1 -> [delta_PLL]
  [CosSinTheta] -> CosSin_Delay2/1
  dq02abc_norm/2 -> Bus Generator4/1, vm_abc_ref_pu/1  "vm_abc_pu"
  Current control/1(vm) -> dq02abc_norm/1, RMS derivation3/1, Bus Generator4/2  "vm_dq"
  vg_abc_pu/1 -> [vg_abc_pu], PLL/1, " pu P/Q computation"/1(v_abc_pu)
  Bus Generator/1 -> [Ig]  "Ig"
  Bus Creator/1 -> Signal Conversion/1
  [Vm] -> Bus Creator/5  "Vm"
  Eq_set/1 -> Mux/2
  [CosSinTheta] -> abc2dq0_norm/2
  abc2dq0_norm/2 -> RMS derivation1/1, Demux/1, Scope/1, [ig_dq]  "ig_dq"
  " pu P/Q computation"/1(P) -> To Workspace/1, [P]  "P"
  Power Control Loops1/1(f) -> [f]  "f"
  [w_PLL] -> Power Control Loops1/4(w_PLL)
  P_set/1 -> Power Control Loops1/2(P_set)
  [delta_PLL] -> Power Control Loops1/3(delta_PLL)
  " pu P/Q computation"/2(Q) -> [Q]  "Q"
  E_set/1 -> Mux/1
  [f] -> Bus Creator/3  "f"
  [Q] -> Bus Creator/2  "Q"
  [P] -> Bus Creator/1  "P"
  Signal Conversion/1 -> m/1
  [idq_unsat] -> Virtual Active Power calculation/2(Current+)
  [vg_dq] -> Virtual Active Power calculation/1(Voltage+)
  Virtual Active Power calculation/1(Virtual Active Power) -> Unit Delay2/1
  Manual Switch/1 -> Power Control Loops1/1(P_mes)
  [VirtualP] -> Scope2/1, Manual Switch/1
  [P] -> Scope2/2, Manual Switch/2
  ig_abc_pu/1 -> abc2dq0_norm/1, Bus Generator/1, " pu P/Q computation"/2(i_abc_pu)  "is_abc_pu"
  [vg_dq] -> Bus Generator2/2, RMS derivation2/1
  Current reference generation/1(Is_dq*) -> [idq_unsat], I_sat2/1(is_dq*+)
  [ig_dq] -> Current control/1(Ig_dq)
  I_sat2/1(is_dq*sat) -> Current control/2(Ig_dq*)
  [vg_dq] -> Current reference generation/2(vg_dq)
  Mux/1 -> Current reference generation/1(Vm_dq*)
  [vg_dq] -> Current control/3(vg_dq)
  [Theta] -> Bus Creator/4
  Power Control Loops1/2(Theta) -> [Theta]  "Theta"
  Unit Delay2/1 -> To Workspace1/1, [VirtualP]
  Demux/1 -> To Workspace2/1
  Demux/2 -> To Workspace3/1
  I_sat2/2(sat) -> Power Control Loops1/5(sat)
  RMS derivation1/1 -> To Workspace4/1  "Ig_RMS"

== system GFM_L_Filter_cc/Generic Voltage Source/ pu P//Q computation ==
  v_abc_pu : Inport  PortDimensions=3
  i_abc_pu : Inport  Port=2  PortDimensions=3
  Demux : Demux  Outputs=3
      settings: DisplayOption=none
  Mux : Mux  Inputs=3
  Product1 : Product  InputSameDT=on  SaturateOnIntegerOverflow=on  OutDataTypeStr=Inherit: Same as first input
  Product3 : Product  InputSameDT=on  SaturateOnIntegerOverflow=on  OutDataTypeStr=Inherit: Same as first input
  Sum : Sum  Inputs=+-  InputSameDT=on  SaturateOnIntegerOverflow=on  OutDataTypeStr=Inherit: Same as first input
  Sum1 : Sum  Inputs=1  InputSameDT=on  SaturateOnIntegerOverflow=on  OutDataTypeStr=Inherit: Same as first input
  Sum4 : Sum  Inputs=1  InputSameDT=on  SaturateOnIntegerOverflow=on  OutDataTypeStr=Inherit: Same as first input
  Sum5 : Sum  Inputs=+-  InputSameDT=on  SaturateOnIntegerOverflow=on  OutDataTypeStr=Inherit: Same as first input
  Sum6 : Sum  Inputs=+-  InputSameDT=on  SaturateOnIntegerOverflow=on  OutDataTypeStr=Inherit: Same as first input
  pu->V : Gain  Gain=1/sqrt(3)  SaturateOnIntegerOverflow=on  OutDataTypeStr=Inherit: Same as input  ParamDataTypeStr=Inherit: Same as input
  pu->V1 : Gain  Gain=1/3  SaturateOnIntegerOverflow=on  OutDataTypeStr=Inherit: Same as input  ParamDataTypeStr=Inherit: Same as input
  pu->V2 : Gain  Gain=1/3  SaturateOnIntegerOverflow=on  OutDataTypeStr=Inherit: Same as input  ParamDataTypeStr=Inherit: Same as input
  p_u : Outport
  q_u : Outport  Port=2
  wires:
  pu->V2/1 -> q_u/1
  pu->V1/1 -> p_u/1
  Sum1/1 -> pu->V/1
  Product3/1 -> Sum1/1
  Product1/1 -> Sum4/1
  v_abc_pu/1 -> Product1/1, Demux/1
  i_abc_pu/1 -> Product1/2, Product3/2
  Sum4/1 -> pu->V1/1
  Demux/1 -> Sum/1, Sum6/2
  Demux/2 -> Sum/2, Sum5/1
  Demux/3 -> Sum5/2, Sum6/1
  Sum/1 -> Mux/3
  Sum5/1 -> Mux/1
  Sum6/1 -> Mux/2
  Mux/1 -> Product3/1
  pu->V/1 -> pu->V2/1  "Q"

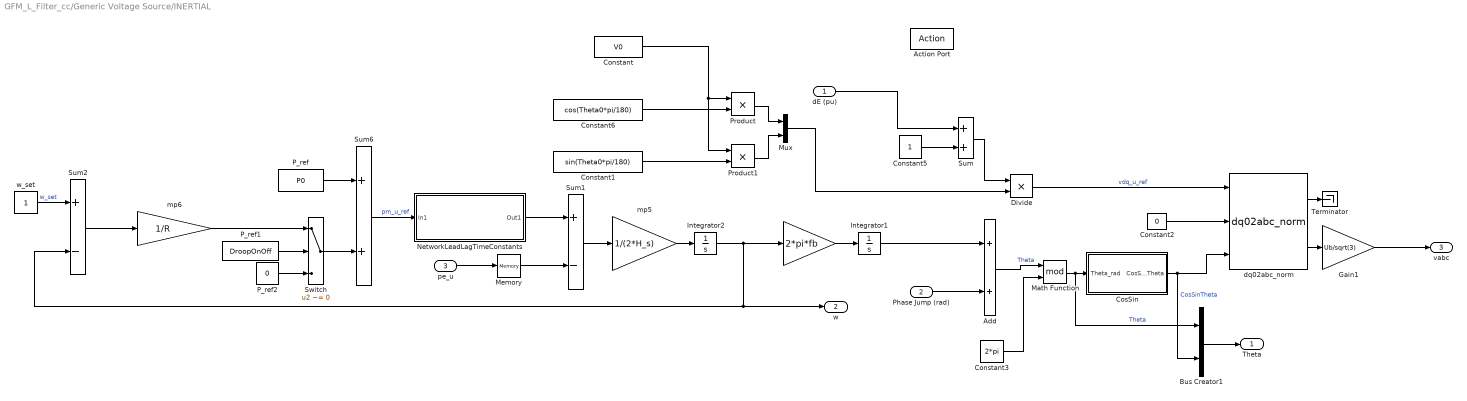
== system GFM_L_Filter_cc/Generic Voltage Source/INERTIAL ==
  dE (pu) : Inport
  Phase Jump (rad) : Inport  Port=2
  pe_u : Inport  Port=3
  Action Port : ActionPort
  " " : Gain  Gain=2*pi*fb
  Add : Sum
  Bus Creator1 : BusCreator  Inputs=2
  Constant : Constant  Value=V0
  Constant1 : Constant  Value=sin(Theta0*pi/180)
  Constant2 : Constant  Value=0
  Constant3 : Constant  Value=2*pi
  Constant5 : Constant
  Constant6 : Constant  Value=cos(Theta0*pi/180)
  CosSin : Subsystem
  Divide : Product  Inputs=**
  Gain1 : Gain  Gain=Ub/sqrt(3)
  Integrator1 : Integrator  InitialCondition=Theta0*pi/180
  Integrator2 : Integrator  InitialCondition=1
  Math Function : Math  Operator=mod  SaturateOnIntegerOverflow=on
  Memory : Memory
  Mux : Mux  Inputs=2
  NetworkLeadLagTimeConstants : Subsystem
  P_ref : Constant  Value=P0
  P_ref1 : Constant  Value=DroopOnOff
  P_ref2 : Constant  Value=0
  Product : Product
  Product1 : Product
  Sum : Sum
  Sum1 : Sum  Inputs=+-
  Sum2 : Sum  Inputs=+-
  Sum6 : Sum
  Switch : Switch  Criteria=u2 ~= 0
  Terminator : Terminator
  dq02abc_norm : Control_Lib/dq02abc_norm  referenceAxisMode=Reference axis at 90 degrees behind phase_a  baseUpdateGain=sqrt(3)
  mp5 : Gain  Gain=1/(2*H_s)
  mp6 : Gain  Gain=1/R
  w_set : Constant
  Theta : Outport
  w : Outport  Port=2
  vabc : Outport  Port=3
  wires:
  Memory/1 -> Sum1/2
  w_set/1 -> Sum2/1  "w_set"
  Switch/1 -> Sum6/2
  Integrator1/1 -> Add/1
  Sum6/1 -> NetworkLeadLagTimeConstants/1(In1)  "pm_u_ref"
  Sum1/1 -> mp5/1
  pe_u/1 -> Memory/1
  mp5/1 -> Integrator2/1
  P_ref1/1 -> Switch/2
  Integrator2/1 -> w/1, Sum2/2, " "/1
  P_ref2/1 -> Switch/3
  Sum2/1 -> mp6/1
  " "/1 -> Integrator1/1
  mp6/1 -> Switch/1
  P_ref/1 -> Sum6/1
  NetworkLeadLagTimeConstants/1(Out1) -> Sum1/1
  Bus Creator1/1 -> Theta/1
  Mux/1 -> Divide/2
  Constant5/1 -> Sum/2
  Product1/1 -> Mux/2
  Constant2/1 -> dq02abc_norm/2
  Math Function/1 -> CosSin/1(Theta_rad), Bus Creator1/1  "Theta"
  Add/1 -> Math Function/1  "Theta"
  Phase Jump (rad)/1 -> Add/2
  Constant/1 -> Product1/1, Product/1
  Divide/1 -> dq02abc_norm/1  "vdq_u_ref"
  Constant1/1 -> Product1/2
  CosSin/1(CosSinTheta) -> dq02abc_norm/3, Bus Creator1/2  "CosSinTheta"
  Constant3/1 -> Math Function/2
  Constant6/1 -> Product/2
  Product/1 -> Mux/1
  Gain1/1 -> vabc/1
  Sum/1 -> Divide/1
  dq02abc_norm/1 -> Terminator/1
  dE (pu)/1 -> Sum/1
  dq02abc_norm/2 -> Gain1/1

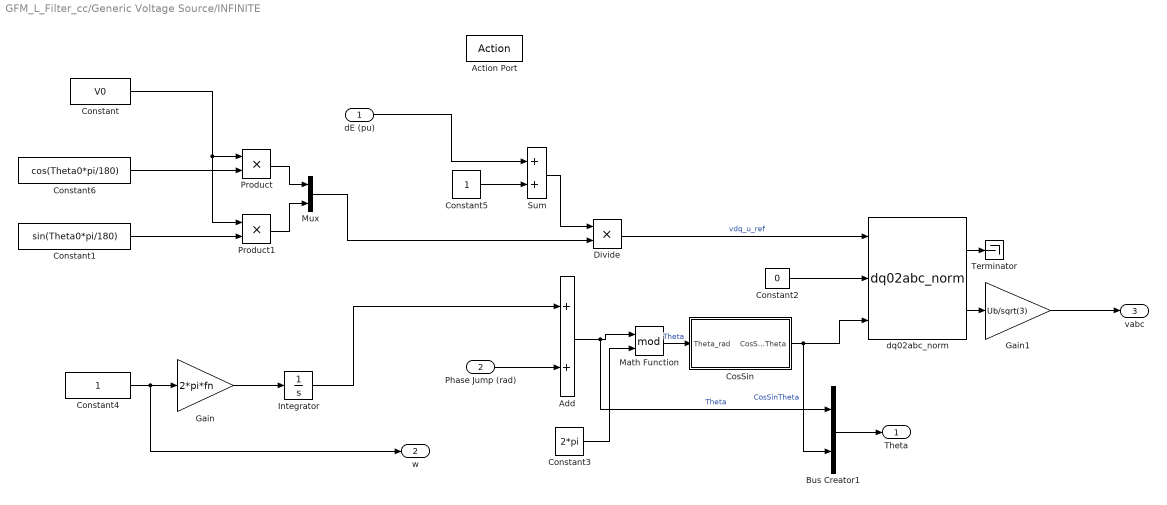
== system GFM_L_Filter_cc/Generic Voltage Source/INFINITE ==
  dE (pu) : Inport
  Phase Jump (rad) : Inport  Port=2
  Action Port : ActionPort
  Add : Sum
  Bus Creator1 : BusCreator  Inputs=2
  Constant : Constant  Value=V0
  Constant1 : Constant  Value=sin(Theta0*pi/180)
  Constant2 : Constant  Value=0
  Constant3 : Constant  Value=2*pi
  Constant4 : Constant
  Constant5 : Constant
  Constant6 : Constant  Value=cos(Theta0*pi/180)
  CosSin : Subsystem
  Divide : Product  Inputs=**
  Gain : Gain  Gain=2*pi*fn
  Gain1 : Gain  Gain=Ub/sqrt(3)
  Integrator : Integrator  InitialCondition=Theta0*pi/180
  Math Function : Math  Operator=mod  SaturateOnIntegerOverflow=on
  Mux : Mux  Inputs=2
  Product : Product
  Product1 : Product
  Sum : Sum
  Terminator : Terminator
  dq02abc_norm : Control_Lib/dq02abc_norm  referenceAxisMode=Reference axis at 90 degrees behind phase_a  baseUpdateGain=sqrt(3)
  Theta : Outport
  w : Outport  Port=2
  vabc : Outport  Port=3
  wires:
  Bus Creator1/1 -> Theta/1
  Mux/1 -> Divide/2
  Constant5/1 -> Sum/2
  Product1/1 -> Mux/2
  Constant2/1 -> dq02abc_norm/2
  Math Function/1 -> CosSin/1(Theta_rad)  "Theta"
  Add/1 -> Bus Creator1/1, Math Function/1  "Theta"
  Phase Jump (rad)/1 -> Add/2
  Constant/1 -> Product1/1, Product/1
  Divide/1 -> dq02abc_norm/1  "vdq_u_ref"
  Constant1/1 -> Product1/2
  CosSin/1(CosSinTheta) -> dq02abc_norm/3, Bus Creator1/2  "CosSinTheta"
  Constant3/1 -> Math Function/2
  Constant6/1 -> Product/2
  Product/1 -> Mux/1
  Gain1/1 -> vabc/1
  Constant4/1 -> Gain/1, w/1
  Sum/1 -> Divide/1
  dq02abc_norm/1 -> Terminator/1
  dE (pu)/1 -> Sum/1
  Gain/1 -> Integrator/1
  Integrator/1 -> Add/1
  dq02abc_norm/2 -> Gain1/1

== system GFM_L_Filter_cc/Generic Voltage Source/Source_For_OP ==
  v_abc_ref : Inport
  Controlled Voltage Source1 : powerlib/Electrical Sources/Controlled Voltage Source  Initialize=off  Source_Type=AC  Amplitude=V0*Ub*sqrt(2/3)*sin(Theta0)  Phase=(Theta0*180/pi)  Frequency=fb  Measurements=None
  Controlled Voltage Source2 : powerlib/Electrical Sources/Controlled Voltage Source  Initialize=off  Source_Type=AC  Amplitude=V0*Ub*sqrt(2/3)*sin(Theta0-2*pi/3)  Phase=(Theta0*180/pi)-120  Frequency=fb  Measurements=None
  Controlled Voltage Source3 : powerlib/Electrical Sources/Controlled Voltage Source  Initialize=off  Source_Type=AC  Amplitude=V0*Ub*sqrt(2/3)*sin(Theta0-4*pi/3)  Phase=(Theta0*180/pi)+120  Frequency=fb  Measurements=None
  Demux : Demux  Outputs=3
  Step : Step  Time=1e-9  SampleTime=0
  Subsystem3 : Subsystem
  Three-Phase Source1 : powerlib/Electrical Sources/Three-Phase Source  InternalConnection=Yn  VoltagePhases=off  Voltage=V0*Ub  PhaseAngle=Theta0  Voltage_phases=[25e3 25e3 25e3]/sqrt(3)  PhaseAngles_phases=[0 -120 +120]  Frequency=fb  NonIdealSource=off  SpecifyImpedance=off  Resistance=0.8929  Inductance=16.58e-3  ShortCircuitLevel=100e6  BaseVoltage=25e3  XRratio=7  BusType=swing  Pref=10e3  Qref=0  Prefabc=[10e3, 10e3, 10e3]  Qrefabc=[0, 0, 0]  Qmin=-inf  Qmax=inf
  A : PMIOPort  Side=Right
  B : PMIOPort  Port=2  Side=Right
  C : PMIOPort  Port=3  Side=Right
  N : PMIOPort  Port=4  Side=Left
  wires:
  Demux/2 -> Controlled Voltage Source2/1
  v_abc_ref/1 -> Demux/1
  Demux/1 -> Controlled Voltage Source1/1
  Demux/3 -> Controlled Voltage Source3/1
  Step/1 -> Subsystem3/1(switch)
  connections:
  Controlled Voltage Source3/LConn1 -- Three-Phase Source1/LConn1 -- N/RConn1 -- Controlled Voltage Source2/LConn1 -- Controlled Voltage Source1/LConn1
  Subsystem3/RConn1 -- A/RConn1
  Subsystem3/RConn2 -- B/RConn1
  Subsystem3/RConn3 -- C/RConn1
  Controlled Voltage Source1/RConn1 -- Subsystem3/LConn1
  Controlled Voltage Source2/RConn1 -- Subsystem3/LConn2
  Controlled Voltage Source3/RConn1 -- Subsystem3/LConn3
  Three-Phase Source1/RConn1 -- Subsystem3/LConn4
  Three-Phase Source1/RConn2 -- Subsystem3/LConn5
  Three-Phase Source1/RConn3 -- Subsystem3/LConn6

== system GFM_L_Filter_cc/GFM_CC IDEAL_VSC/Control loops2/ pu P//Q computation ==
  v_abc_pu : Inport  PortDimensions=3
  i_abc_pu : Inport  Port=2  PortDimensions=3
  Demux : Demux  Outputs=3
      settings: DisplayOption=none
  Mux : Mux  Inputs=3
  Product1 : Product  InputSameDT=on  SaturateOnIntegerOverflow=on  OutDataTypeStr=Inherit: Same as first input
  Product3 : Product  InputSameDT=on  SaturateOnIntegerOverflow=on  OutDataTypeStr=Inherit: Same as first input
  Sum : Sum  Inputs=+-  InputSameDT=on  SaturateOnIntegerOverflow=on  OutDataTypeStr=Inherit: Same as first input
  Sum1 : Sum  Inputs=1  InputSameDT=on  SaturateOnIntegerOverflow=on  OutDataTypeStr=Inherit: Same as first input
  Sum4 : Sum  Inputs=1  InputSameDT=on  SaturateOnIntegerOverflow=on  OutDataTypeStr=Inherit: Same as first input
  Sum5 : Sum  Inputs=+-  InputSameDT=on  SaturateOnIntegerOverflow=on  OutDataTypeStr=Inherit: Same as first input
  Sum6 : Sum  Inputs=+-  InputSameDT=on  SaturateOnIntegerOverflow=on  OutDataTypeStr=Inherit: Same as first input
  pu->V : Gain  Gain=1/sqrt(3)  SaturateOnIntegerOverflow=on  OutDataTypeStr=Inherit: Same as input  ParamDataTypeStr=Inherit: Same as input
  pu->V1 : Gain  Gain=1/3  SaturateOnIntegerOverflow=on  OutDataTypeStr=Inherit: Same as input  ParamDataTypeStr=Inherit: Same as input
  pu->V2 : Gain  Gain=1/3  SaturateOnIntegerOverflow=on  OutDataTypeStr=Inherit: Same as input  ParamDataTypeStr=Inherit: Same as input
  P : Outport
  Q : Outport  Port=2
  wires:
  pu->V2/1 -> Q/1
  pu->V1/1 -> P/1
  Sum1/1 -> pu->V/1
  Product3/1 -> Sum1/1
  Product1/1 -> Sum4/1
  v_abc_pu/1 -> Product1/1, Demux/1
  i_abc_pu/1 -> Product1/2, Product3/2
  Sum4/1 -> pu->V1/1
  Demux/1 -> Sum/1, Sum6/2
  Demux/2 -> Sum/2, Sum5/1
  Demux/3 -> Sum5/2, Sum6/1
  Sum/1 -> Mux/3
  Sum5/1 -> Mux/1
  Sum6/1 -> Mux/2
  Mux/1 -> Product3/1
  pu->V/1 -> pu->V2/1  "Q"

== system GFM_L_Filter_cc/GFM_CC IDEAL_VSC/Control loops2/Current control ==
  Ig_dq : Inport
  Ig_dq* : Inport  Port=2
  vg_dq : Inport  Port=3
  Constant : Constant
  Current control : Subsystem
  vm : Outport  InitialOutput=0
  wires:
  Constant/1 -> Current control/4(w)
  Ig_dq/1 -> Current control/1(Is_dq)
  Ig_dq*/1 -> Current control/3(Is_dq_ref)
  vg_dq/1 -> Current control/2(Eg_dqfr)
  Current control/1(vm_dq_ref) -> vm/1
